simulink model "LQR_sim_vel"  (R2025b)
settings: Solver=VariableStepAuto  StartTime=0.0  StopTime=5  RelTol=1e-3
undefined symbols (not defined in the file): A, B, C, D, ic, K, Kr
settings Model: Creator=JPham  LastModifiedBy=JPham

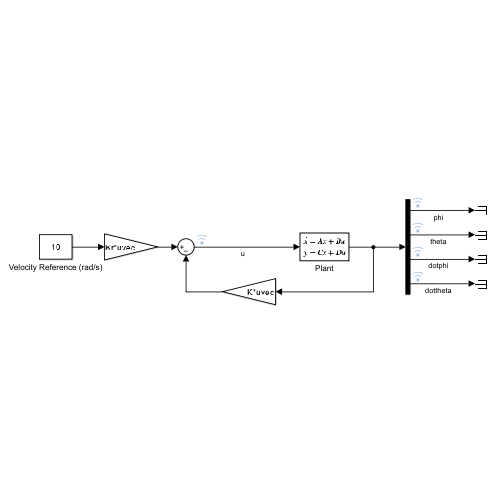
[thumbnail: Simulink's stored preview of the top-level diagram]
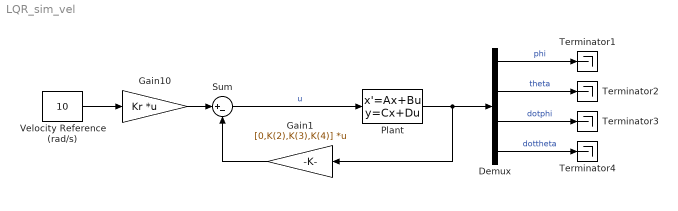
== system LQR_sim_vel ==
  Demux : Demux
  Gain1 : Gain  Gain=[0,K(2),K(3),K(4)]  Multiplication=Matrix(K*u) (u vector)
  Gain10 : Gain  Gain=Kr  Multiplication=Matrix(K*u) (u vector)
  Plant : StateSpace  A=A  B=B  C=C  D=D  InitialCondition=ic  ContinuousStateAttributes={'phi', 'theta', 'dot_phi', 'dot_theta'}
  Sum : Sum  Inputs=|+-
  Terminator{1..4} (4 alike) : Terminator
  Velocity Reference (rad/s) : Constant  Value=10
  wires:
  Demux/3 -> Terminator3/1  "dotphi"
  Velocity Reference (rad/s)/1 -> Gain10/1
  Demux/2 -> Terminator2/1  "theta"
  Gain10/1 -> Sum/1
  Demux/1 -> Terminator1/1  "phi"
  Sum/1 -> Plant/1  "u"
  Demux/4 -> Terminator4/1  "dottheta"
  Gain1/1 -> Sum/2
  Plant/1 -> Gain1/1, Demux/1
